simulink model "sim"  (R2024b)
settings: Solver=VariableStepAuto  StartTime=0.0  StopTime=10.0  RelTol=1e-3
values from neighbouring files (symbols this model uses):
  d = 2    [mFile.m]
  F = 1    [mFile.m]
  k = 3    [mFile.m]
  m1 = 7    [mFile.m]
  m2 = 4    [mFile.m]
settings Model: Creator=Ishak  LastModifiedBy=Ishak

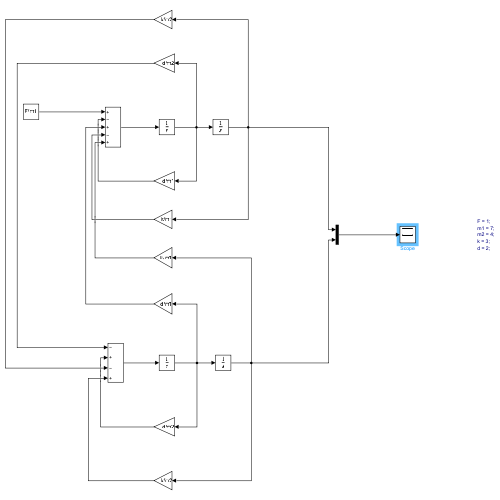
[thumbnail: Simulink's stored preview of the top-level diagram]
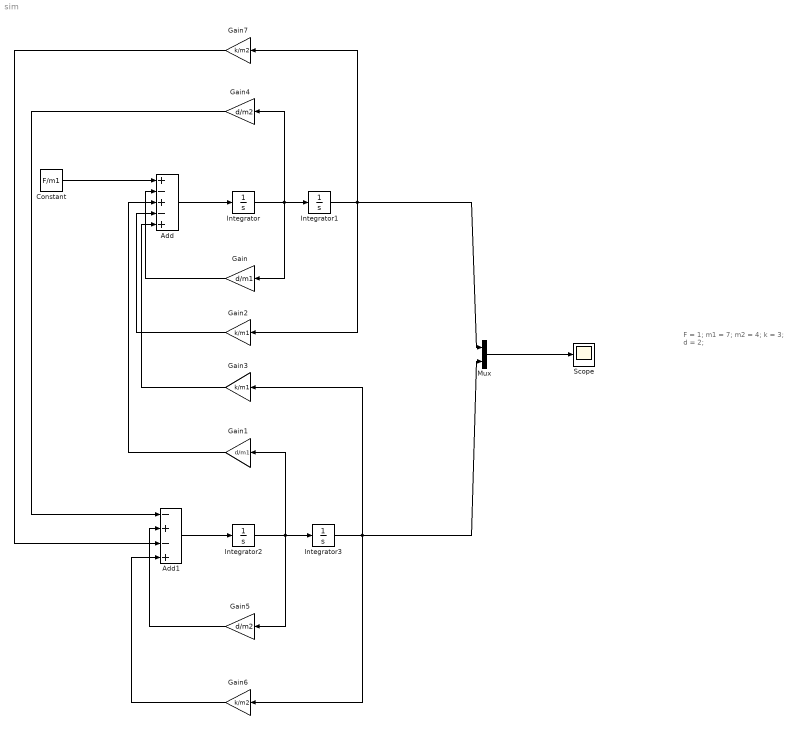
== system sim ==
  note: F = 1;
      | m1 = 7;
      | m2 = 4;
      | k = 3;
      | d = 2;
  Add : Sum  Inputs=+-+-+
  Add1 : Sum  Inputs=-+-+
  Constant : Constant  Value=F/m1
  Gain : Gain  Gain=d/m1
  Gain1 : Gain  Gain=d/m1
  Gain2 : Gain  Gain=k/m1
  Gain3 : Gain  Gain=k/m1
  Gain4 : Gain  Gain=d/m2
  Gain5 : Gain  Gain=d/m2
  Gain6 : Gain  Gain=k/m2
  Gain7 : Gain  Gain=k/m2
  Integrator{,1..3} (4 alike) : Integrator
  Mux : Mux  Inputs=2
  Scope : Scope
  wires:
  Integrator1/1 -> Gain2/1, Mux/1, Gain7/1
  Add/1 -> Integrator/1
  Integrator/1 -> Gain4/1, Gain/1, Integrator1/1
  Constant/1 -> Add/1
  Gain/1 -> Add/2
  Integrator2/1 -> Gain5/1, Gain1/1, Integrator3/1
  Integrator3/1 -> Gain3/1, Mux/2, Gain6/1
  Add1/1 -> Integrator2/1
  Gain1/1 -> Add/3
  Gain2/1 -> Add/4
  Gain3/1 -> Add/5
  Gain4/1 -> Add1/1
  Gain5/1 -> Add1/2
  Gain6/1 -> Add1/4
  Gain7/1 -> Add1/3
  Mux/1 -> Scope/1
